simulink model "SAD_project"  (R2019a)
settings: Solver=FixedStepAuto  StartTime=0.0  StopTime=inf  FixedStep=1e-3  RelTol=1e-3  EnableMultiTasking=on
libraries: arduinosensorlib x1
settings Model: SimulationMode=external  ExtModeTrigDuration=2  Creator=morsh  LastModifiedBy=morsh
settings OptimizationCC: EnhancedBackFolding=on  PassReuseOutputArgsAs=Individual arguments  MaxStackSize=64  OptimizeBlockOrder=speed  DifferentSizesBufferReuse=on  OptimizationCustomize=off
settings DebuggingCC: ParameterTunabilityLossMsg=error
settings HardwareCC: ProdBitPerInt=16  ProdBitPerPointer=16  ProdBitPerSizeT=16  ProdBitPerPtrDiffT=16  ProdLargestAtomicFloat=None  ProdWordSize=8  ProdHWDeviceType=Atmel->AVR  UseEmbeddedCoderFeatures=off
settings SFSimCC: MATLABDynamicMemAlloc=off
settings RTWCC: SystemTargetFile=ert.tlc  HardwareBoard=Arduino Mega 2560  TLCOptions=-aInlineSetEventsForThisBaseRateFcn=TLC_FALSE -aSuppressMultiTaskScheduler=TLC_FALSE -aRateBasedStepFcn=1  TemplateMakefile=ert_default_tmf  GenerateReport=on  Toolchain=Arduino AVR  BuildConfiguration=Faster Runs  IncludeHyperlinkInReport=on  LaunchReport=on  GenerateTraceInfo=on  GenerateTraceReport=on  GenerateTraceReportSl=on  GenerateTraceReportSf=on  GenerateTraceReportEml=on
settings CodeAppCC: ForceParamTrailComments=on  IgnoreCustomStorageClasses=off  OperatorAnnotations=on  SimulinkDataObjDesc=on  SFDataObjDesc=on  InsertBlockDesc=on
settings ERTTargetCC: SupportContinuousTime=on  SupportNonInlinedSFcns=on  SupportVariableSizeSignals=on  ExtModeStaticAllocSize=2048

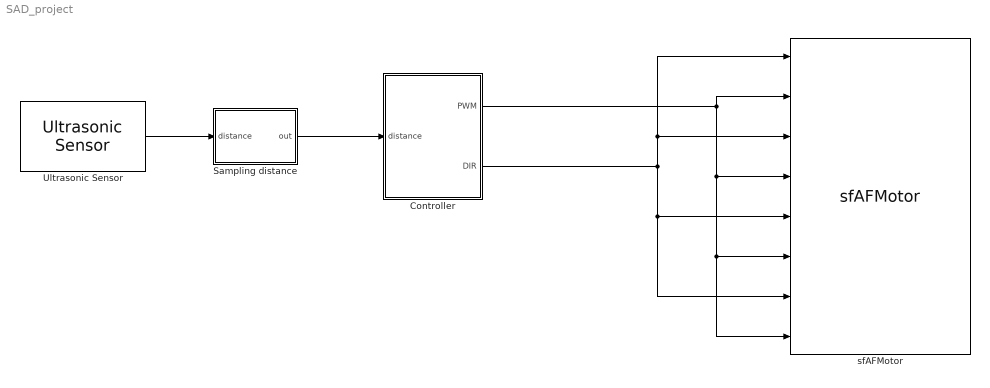
== system SAD_project ==
  Controller : Stateflow chart  BlockKeywords=__PRM__SERIALIZED__DATA__:Stateflow Chart,Stateflow Diagram  TreatAsAtomicUnit=on
  Sampling distance : Stateflow chart  BlockKeywords=__PRM__SERIALIZED__DATA__:Stateflow Chart,Stateflow Diagram  TreatAsAtomicUnit=on
  Ultrasonic Sensor : arduinosensorlib/Ultrasonic Sensor  NumSignalPins=2  TrigPin=51  EchoPin=50  SignalPin=3  SampleTime_=-1  blockPlatform=ARDUINO
      settings: SourceProductName=Simulink Support Package for Arduino Hardware  SourceProductBaseCode=ARDUINO
  sfAFMotor : S-Function  InitFcn=try, set_param(gcb,'FunctionName','sfAFMotor'), end  FunctionName=sfAFMotor  SFunctionModules=sfAFMotor_wrapper  SFunctionDeploymentMode=off  EnableBusSupport=off  mask(S-Function Builder){}
      mask help: Simulink:masks:SFunctionBuilder_MD
      mask init:
      | val = [[.9  0.75 0.75 1 1 .9 .9 1]',[1 1 0.75 0.75 .9 .9 1 .9]'];try , sys = get_param(gcb,'SfunBuilderFcnName');if isempty(sys), sys = get_param(gcb,'FunctionName'); end,catch, sys = get_param(gcb,'FunctionName'); end
      settings: CopyFcn=set_param(gcbh,'LinkStatus','none')  PreSaveFcn=try, set_param(gcb,'FunctionName','sfAFMotor'), end  OpenFcn=sfunctionwizard(gcbh)
      mask Display:
      | plot(val(:,1),val(:,2))
      | disp(sys)
      | port_label('input',1,'DIR1')
      | port_label('input',2,'PWM1')
      | port_label('input',3,'DIR2')
      | port_label('input',4,'PWM2')
      | port_label('input',5,'DIR3')
      | port_label('input',6,'PWM3')
      | port_label('input',7,'DIR4')
      | port_label('input',8,'PWM4')
  wires:
  Controller/2(DIR) -> sfAFMotor/7, sfAFMotor/5, sfAFMotor/3, sfAFMotor/1
  Controller/1(PWM) -> sfAFMotor/2, sfAFMotor/4, sfAFMotor/6, sfAFMotor/8
  Ultrasonic Sensor/1 -> Sampling distance/1(distance)
  Sampling distance/1(out) -> Controller/1(distance)

== stateflow chart SAD_project/Sampling distance ==
  state value
    entry:
    v1=distance;
  state value2
    entry:
    out=v1;
  (default) -> value
  value -> value2
  value2 -> value : [after(0.1,sec)]
  data: v1 local; out output; distance input

== stateflow chart SAD_project/Controller ==
  state Backward
    entry:
    DIR=2;
  state stop
    entry:
    PWM=0;
    DIR=3;
  state Forward
    entry:
    DIR=1;
  state Add
    entry:
    PWM=(PWM+1);
    q=0;
    if(p==1 && distance<0.2)
    q=1;
    end
    if(p==2 && distance>=0.2)
    q=1;
    end
  (default) -> stop
  Backward -> stop [order 1] : [distance>=0.2]
  Forward -> stop [order 2] : [distance<0.2]
  Add -> Backward [order 4] : [PWM==255 && p==2]{flag=1}
  stop -> Backward [order 2] : [distance<0.2]{flag=0}
  stop -> Forward [order 1] : [distance>=0.2]{flag=0}
  Add -> Forward [order 3] : [PWM==255 && p==1]{flag=1}
  Backward -> Add [order 2] : [flag~=1]{PWM=0, p=2}
  Add -> stop [order 5] : [distance>=0.2 && p==2]
  Add -> stop [order 1] : [distance<0.2 && p==1]
  Forward -> Add [order 1] : [flag~=1]{PWM=0, p=1}
  Add -> Add [order 2] : [after(0.01,sec) && PWM~= 255 && q==0]
  data: PWM output uint8; DIR output uint8; distance input double; flag local; p local; q local; z local
